simulink model "model7_video_qpsk_ofdm"  (R2025b)
settings: Solver=FixedStepDiscrete  StartTime=0.0  StopTime=1  RelTol=1e-3
values from neighbouring files (symbols this model uses):
  txFrameBits = double(txFrameBits(:))    [reconstruct_video_frames.m]    (also in setup_simulink_streaming_coded_const.m = [preambleBits; txCodedBitsPadded])
libraries: commofdm x2, commdigbbndpm3 x2, commchan3 x1
settings Model: Creator=Naren  LastModifiedBy=Naren

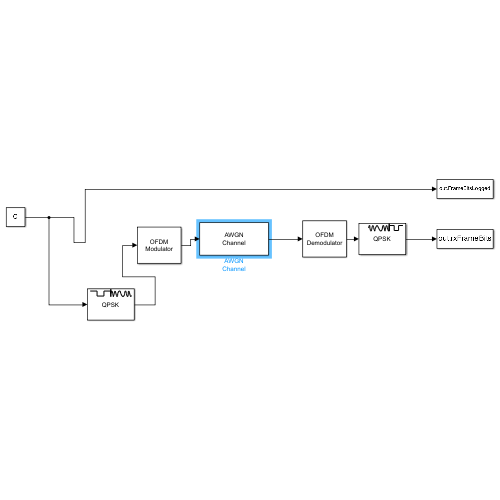
[thumbnail: Simulink's stored preview of the top-level diagram]
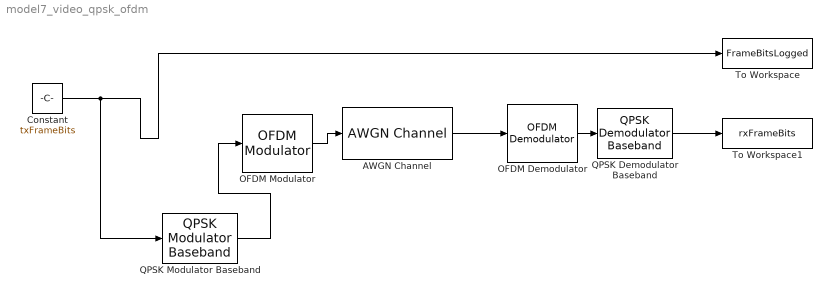
== system model7_video_qpsk_ofdm ==
  AWGN Channel : commchan3/AWGN Channel  LegacyMode=off  NoiseMethod="Signal to noise ratio  (SNR)"  noiseMode="Signal to noise ratio  (SNR)"  EbNo=10  EsNo=10  SNR=60  BitsPerSymbol=1  SignalPower=1  SpecifySymbolPeriod=off  SamplesPerSymbol=1  SymbolPeriod=1  VarianceSource=Parameter  Variance=1  RandomStream=Global stream  Seed=67  SimulateUsing=Code generation
  Constant : Constant  Value=txFrameBits
  OFDM Demodulator : commofdm/OFDM Demodulator  StatePerturbationForJacobian=1.0e-05  FFTLength=64  NumGuardBandCarriers=[7; 8]  RemoveDCCarrier=on  PilotOutputPort=off  PilotCarrierIndices=[12; 26; 40; 54]  CyclicPrefixLength=16  OversamplingFactor=1  NumSymbols=1  NumReceiveAntennas=1  SimulateUsing=Interpreted execution
  OFDM Modulator : commofdm/OFDM Modulator  StatePerturbationForJacobian=1.0e-05  FFTLength=64  NumGuardBandCarriers=[7; 8]  InsertDCNull=on  PilotInputPort=off  PilotCarrierIndices=[12; 26; 40; 54]  CyclicPrefixLength=16  Windowing=off  WindowLength=1  OversamplingFactor=1  NumSymbols=1  NumTransmitAntennas=1  SimulateUsing=Interpreted execution
  QPSK Demodulator Baseband : commdigbbndpm3/QPSK Demodulator Baseband  OutType=Bit  DecType=Hard decision  VarSource=Dialog  Variance=1  Dec=Gray  Ph=pi/4  outDtype1=Inherit via internal rule  outDtype2=Inherit via internal rule  derotateFactorWordLen=16  derotateFactorDataTypeStr=Inherit: Same word length as input  derotateFactorLastDataTypeStr=Inherit: Same word length as input
  QPSK Modulator Baseband : commdigbbndpm3/QPSK Modulator Baseband  InType=Bit  Enc=Gray  Ph=pi/4  outDtype=double  outWordLen=16  outUDDataType=sfix(16)  outFracLenMode=Best precision  outFracLen=15  outDataTypeStr=double  outLastDataTypeStr=double
  To Workspace : ToWorkspace  VariableName=FrameBitsLogged  SampleTime=-1
  To Workspace1 : ToWorkspace  VariableName=rxFrameBits  SampleTime=-1
  wires:
  AWGN Channel/1 -> OFDM Demodulator/1
  QPSK Demodulator Baseband/1 -> To Workspace1/1
  QPSK Modulator Baseband/1 -> OFDM Modulator/1
  OFDM Modulator/1 -> AWGN Channel/1
  OFDM Demodulator/1 -> QPSK Demodulator Baseband/1
  Constant/1 -> QPSK Modulator Baseband/1, To Workspace/1
